simulink model "neural_network_based_adaptive_sliding"  (R2017b)
settings: Solver=ode45  StartTime=0  StopTime=20  RelTol=1e-3
undefined symbols (not defined in the file or in its folder): sigbuilder_block
libraries: simulink x2
settings Model: Creator=Melik  LastModifiedBy=Melik

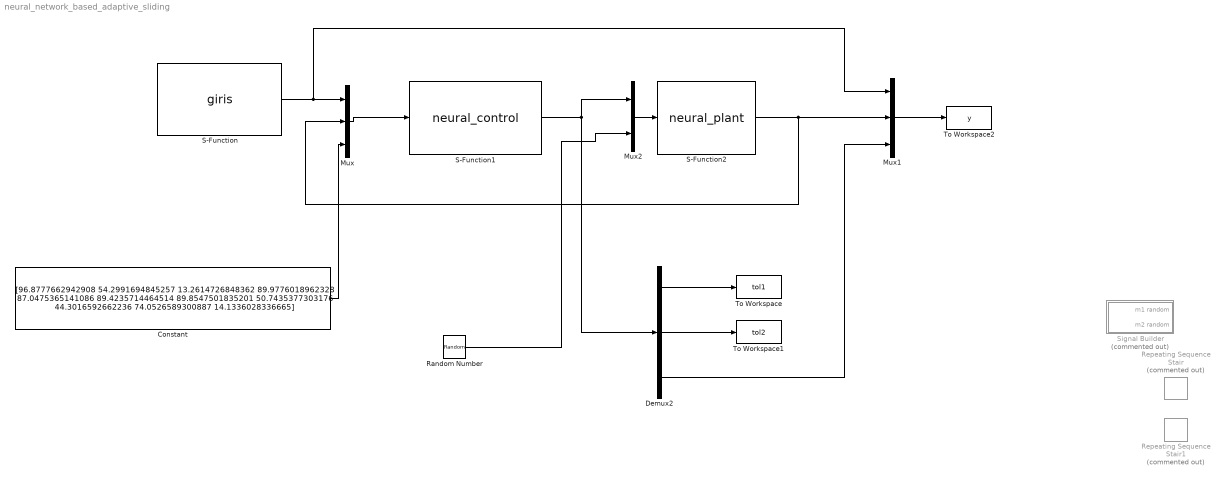
== system neural_network_based_adaptive_sliding ==
  Constant : Constant  Value=[96.8777662942908 54.2991694845257 13.2614726848362 89.9776018962328 87.0475365141086 89.4235714464514 89.8547501835201 50.7435377303176 44.3016592662236 74.0526589300887 14.1336028336665]
  Demux2 : Demux  Outputs=3
  Mux : Mux  Inputs=3
  Mux1 : Mux  Inputs=3
  Mux2 : Mux  Inputs=2
  Random Number : RandomNumber  Variance=0.12  SampleTime=0.1
  Repeating Sequence Stair : simulink/Sources/Repeating Sequence Stair  Commented=on  OutValues=[1.1 1.1 1 1 1 0.9 1.1 1.1 1 1]  tsamp=1  OutMin=[]  OutMax=[]  OutDataTypeStr=double  OutputDataTypeScalingMode=double  OutDataType=fixdt(0,8)  ConRadixGroup=Best Precision: Vector-wise  OutScaling=2^-12
  Repeating Sequence Stair1 : simulink/Sources/Repeating Sequence Stair  Commented=on  OutValues=[0.55 0.55 0.5 0.5 0.5 0.45 0.55 0.55 0.5 0.5]  tsamp=1  OutMin=[]  OutMax=[]  OutDataTypeStr=double  OutputDataTypeScalingMode=double  OutDataType=fixdt(0,8)  ConRadixGroup=Best Precision: Vector-wise  OutScaling=2^-12
  S-Function : S-Function  FunctionName=giris  SFunctionDeploymentMode=off  EnableBusSupport=off
  S-Function1 : S-Function  FunctionName=neural_control  SFunctionDeploymentMode=off  EnableBusSupport=off
  S-Function2 : S-Function  FunctionName=neural_plant  SFunctionDeploymentMode=off  EnableBusSupport=off
  Signal Builder : Subsystem  Tag=STV Subsys  Commented=on  LoadFcn=sigbuilder_block('load');  StartFcn=sigbuilder_block('start');  StopFcn=sigbuilder_block('stop');  ClipboardFcn=sigbuilder_block('clipboard');  mask(Sigbuilder block){tuvar=[0:10]}
      mask help: Simulink:masks:SigbuilderBlock_MD
      mask init:
      | if ~strcmp(get_param(bdroot(gcbh),'SimulationStatus'),'stopped') tuvar = sigbuilder_block('maskInit'); end
      settings: CopyFcn=sigbuilder_block('copy');  DeleteFcn=sigbuilder_block('delete');  ModelCloseFcn=sigbuilder_block('modelClose');  PreSaveFcn=sigbuilder_block('preSave');  PauseFcn=sigbuilder_block('pause');  ContinueFcn=sigbuilder_block('continue');  NameChangeFcn=sigbuilder_block('namechange');  OpenFcn=sigbuilder_block('open',[-802.5 157.5 550.5 399.75 ]);  CloseFcn=sigbuilder_block('close');
      mask Display: plot(0, 0, 100, 100,[2, 2, 32, 32, 2], [68, 8, 8, 68, 68],[32, 2], [38, 38], [32, 19, 2],[53, 60, 44], [32, 17, 17, 2],[16, 16, 31, 31]);txt = getActiveGroup(gcbh);text(2, 100, txt,'verticalAlignment', 'top');
  To Workspace : ToWorkspace  VariableName=tol1  SaveFormat=Timeseries  SampleTime=-1
  To Workspace1 : ToWorkspace  VariableName=tol2  SaveFormat=Timeseries  SampleTime=-1
  To Workspace2 : ToWorkspace  VariableName=y  SaveFormat=Timeseries  SampleTime=-1
  wires:
  S-Function/1 -> Mux1/1, Mux/1
  Mux/1 -> S-Function1/1
  S-Function1/1 -> Demux2/1, Mux2/1
  S-Function2/1 -> Mux1/2, Mux/2
  Demux2/1 -> To Workspace/1
  Demux2/2 -> To Workspace1/1
  Demux2/3 -> Mux1/3
  Mux1/1 -> To Workspace2/1
  Random Number/1 -> Mux2/2
  Mux2/1 -> S-Function2/1
  Constant/1 -> Mux/3

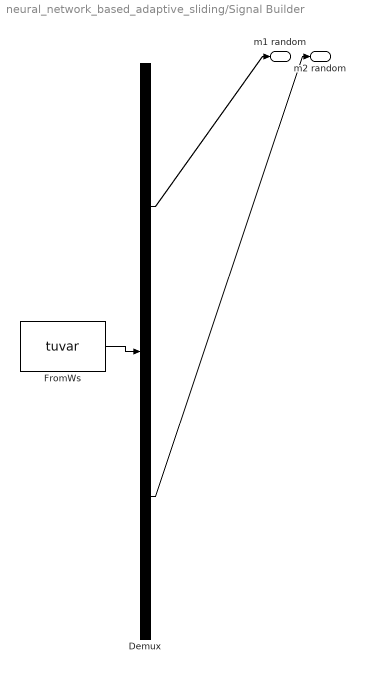
== system neural_network_based_adaptive_sliding/Signal Builder ==
  Demux : Demux  Tag=STV Demux  Outputs=2
  FromWs : FromWorkspace  Tag=STV FromWs  VariableName=tuvar  SampleTime=0
      SigBuilderData=|
      | common.afterFinalStr = 'Extrapolate'
      | common.sampleTime = 0
      | dataSet.timeRange = [0 20]
      | dataSet.name = 'Group 1'
      | sbobj.Groups.Name = 'Group 1'
      | sbobj.Groups.Signals(1).Name = 'm1 random'
      | sbobj.Groups.Signals(1).XData = [0 2 2 5 5 8 8 13 13 18 18 20]
      | sbobj.Groups.Signals(1).YData = [1.1 1.1 1 1 0.9 0.9 1.1 1.1 1 1 0.9 0.9]
      | sbobj.Groups.Signals(2).Name = 'm2 random'
      | sbobj.Groups.Signals(2).XData = [0 2.05 2.05 5 5 8 8 13 13 18 18 20]
      | sbobj.Groups.Signals(2).YData = [0.55 0.55 0.5 0.5 0.45 0.45 0.55 0.55 0.5 0.5 0.45 0.45]
      | sbobj.Groups.TimeRange = [0 20]
  m1 random : Outport  Tag=STV Outport
  m2 random : Outport  Tag=STV Outport  Port=2
  wires:
  FromWs/1 -> Demux/1
  Demux/1 -> m1 random/1
  Demux/2 -> m2 random/1
